simulink model "ex14impsliding4"  (R2025b)
settings: Solver=VariableStepAuto  StartTime=0.0  StopTime=250  RelTol=1e-3
values from neighbouring files (symbols this model uses):
  IJ = inv(J)    [ex16.m]
  J = diag([7000,5900,9600])    [ex16.m]
  q0 = [1;0;0;0]    [ex16.m]
  w0 = [0;0;0]    [ex16.m]
  wr = [1;0;0]    [ex16.m]
libraries: vrlib x1
settings Model: Creator=Esteban  LastModifiedBy=Esteban

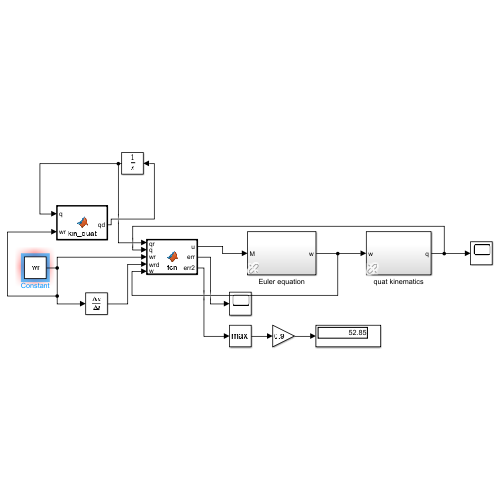
[thumbnail: Simulink's stored preview of the top-level diagram]
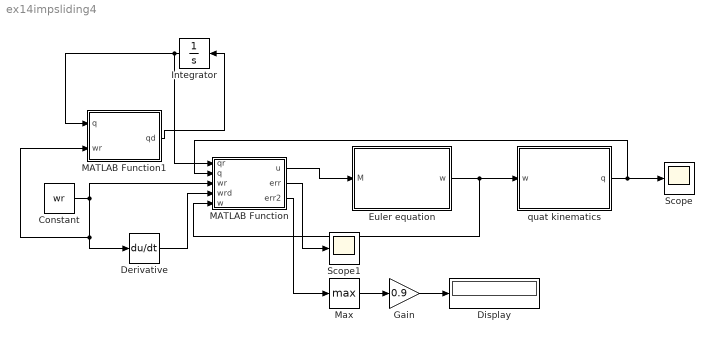
== system ex14impsliding4 ==
  Constant : Constant  Value=wr
  Derivative : Derivative
  Display : Display
  Euler equation : Subsystem  AncestorBlock=lib_rotations_2014/Euler equation
  Gain : Gain  Gain=0.9
  Integrator : Integrator  InitialCondition=[1;0;0;0]
  MATLAB Function : MATLAB Function  TreatAsAtomicUnit=on
  MATLAB Function1 : MATLAB Function  TreatAsAtomicUnit=on
  Max : MinMax  Function=max
  Scope : Scope
      settings: ActiveDisplayYMinimum=-1.5755917816955831  ActiveDisplayYMaximum=1.4631735665723062
  Scope1 : Scope
      settings: ActiveDisplayYMinimum=-0.0021249388111345166  ActiveDisplayYMaximum=0.0052993007032312873
  quat kinematics : Subsystem  AncestorBlock=lib_rotations_2014/quat kinematics
  wires:
  quat kinematics/1(q) -> MATLAB Function/2(q), Scope/1
  Euler equation/1(w) -> MATLAB Function/5(w), quat kinematics/1(w)
  MATLAB Function/1(u) -> Euler equation/1(M)
  MATLAB Function1/1(qd) -> Integrator/1
  Integrator/1 -> MATLAB Function/1(qr), MATLAB Function1/1(q)
  Constant/1 -> MATLAB Function1/2(wr), Derivative/1, MATLAB Function/3(wr)
  Derivative/1 -> MATLAB Function/4(wrd)
  MATLAB Function/2(err) -> Scope1/1
  MATLAB Function/3(err2) -> Max/1
  Max/1 -> Gain/1
  Gain/1 -> Display/1

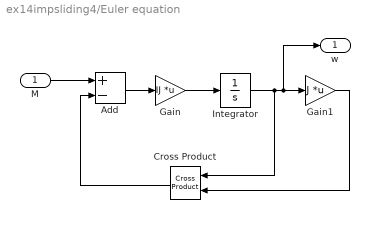
== system ex14impsliding4/Euler equation ==
  M : Inport
  Add : Sum  Inputs=+-
  Cross Product : vrlib/Utilities/Cross Product
  Gain : Gain  Gain=IJ  Multiplication=Matrix(K*u)
  Gain1 : Gain  Gain=J  Multiplication=Matrix(K*u)
  Integrator : Integrator  InitialCondition=w0
  w : Outport  VectorParamsAs1DForOutWhenUnconnected=off
  wires:
  Cross Product/1 -> Add/2
  Add/1 -> Gain/1
  Gain1/1 -> Cross Product/2
  Gain/1 -> Integrator/1
  Integrator/1 -> Gain1/1, w/1, Cross Product/1
  M/1 -> Add/1

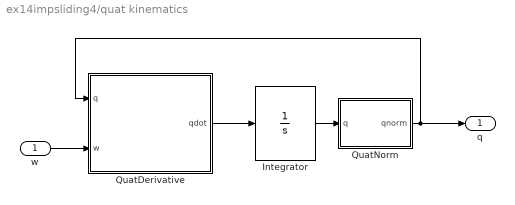
== system ex14impsliding4/quat kinematics ==
  w : Inport  PortDimensions=3
  Integrator : Integrator  InitialCondition=q0
  QuatDerivative : MATLAB Function  TreatAsAtomicUnit=on
  QuatNorm : MATLAB Function  TreatAsAtomicUnit=on
  q : Outport  PortDimensions=4  VectorParamsAs1DForOutWhenUnconnected=off
  wires:
  w/1 -> QuatDerivative/2(w)
  QuatDerivative/1(qdot) -> Integrator/1
  QuatNorm/1(qnorm) -> QuatDerivative/1(q), q/1
  Integrator/1 -> QuatNorm/1(q)

== matlab function ex14impsliding4/quat kinematics/QuatDerivative ==
  data: q input; qdot output; w input
function qdot= QuatDerivative(q,w)
%#codegen
omegaq=[0; w];
Q=[q(1) -q(2) -q(3) -q(4);
    q(2) q(1) -q(4) q(3);
    q(3) q(4) q(1) -q(2);
    q(4) -q(3) q(2) q(1)];
qdot=Q*omegaq/2;

== matlab function ex14impsliding4/quat kinematics/QuatNorm ==
  data: q input; qnorm output
function qnorm = QuatNorm(q)
%#codegen
qnorm=zeros(4,1);
q2=sqrt(q'*q);
qnorm=q/q2;

== matlab function ex14impsliding4/MATLAB Function ==
  data: qr input; u output; q input; wr input; wrd input; w input; err output; err2 output
function [u,err,err2] = fcn(qr,q,wr,wrd,w)

J = diag([7000,5900,9600]);
k1 = 22;
k2 = 196;
n = 1;

qs = [q(1);-q(2:4)];
dq = quatprod(qs,qr);

err = norm(dq(2:4));

dw = wr - w;

us = J*(wrd+(k2/2)*(dq(1)*dw+cross(dq(2:4),wr+w)))+cross(w,J*w);

s = dw + k2*sign(dq(1))*dq(2:4);

u = us + k1*J*tanh(n*s);

err2 = norm(u);

== matlab function ex14impsliding4/MATLAB Function1 ==
  data: q input; qd output; wr input
function qd=kin_quat(q,wr)

% w=[0.2*sin(t);
%     0.5*sin(2*t);
%     0];

q=q/norm(q);

Q=[-q(2) -q(3) -q(4)
    q(1) -q(4) q(3)
    q(4) q(1)  -q(2)
    -q(3) q(2) q(1)];

qd=1/2*Q*wr;
